simulink model "Cim_Motor_Model"  (R2018b)
settings: Solver=VariableStepAuto  StartTime=0.0  StopTime=10.0  RelTol=1e-3
settings Model: Creator=hanso  LastModifiedBy=hanso

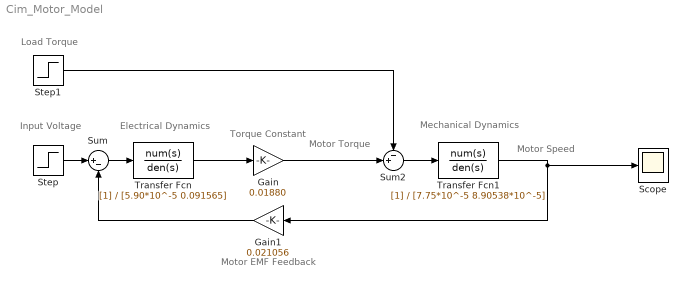
== system Cim_Motor_Model ==
  note: Load Torque
  note: Input Voltage
  note: Mechanical Dynamics
  note: Electrical Dynamics
  note: Torque Constant
  note: Motor EMF Feedback
  note: Motor Speed
  note: Motor Torque
  Gain : Gain  Gain=0.01880
  Gain1 : Gain  Gain=0.021056
  Scope : Scope
  Step : Step  Time=0  After=12  SampleTime=0
  Step1 : Step  SampleTime=0
  Sum : Sum  Inputs=|+-
  Sum2 : Sum  Inputs=-+|
  Transfer Fcn : TransferFcn  Denominator=[5.90*10^-5 0.091565]
  Transfer Fcn1 : TransferFcn  Denominator=[7.75*10^-5 8.90538*10^-5]
  wires:
  Step/1 -> Sum/1
  Sum/1 -> Transfer Fcn/1
  Transfer Fcn/1 -> Gain/1
  Gain/1 -> Sum2/2
  Transfer Fcn1/1 -> Scope/1, Gain1/1
  Gain1/1 -> Sum/2
  Sum2/1 -> Transfer Fcn1/1
  Step1/1 -> Sum2/1
